simulink subsystem "PowerGain"  (R2023a)
settings: Solver=VariableStepAuto  StartTime=0.0  StopTime=10.0  RelTol=1e-3
model mask{Ku=7.27}
  mask prompts: Ku "Коэффициент усиления"
settings Model: Creator=desire  LastModifiedBy=User

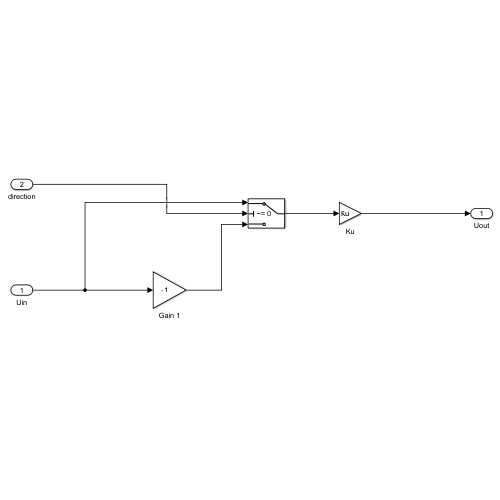
[thumbnail: Simulink's stored preview of the top-level diagram]
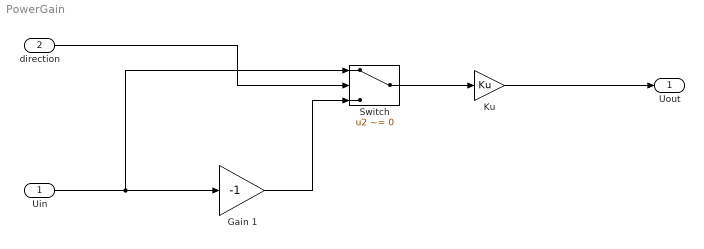
== system PowerGain ==
  Uin : Inport  OutMin=[0]  OutMax=[3.3]
  direction : Inport  Port=2
  Gain 1 : Gain  Gain=-1
  Ku : Gain  Gain=Ku
  Switch : Switch  Criteria=u2 ~= 0  SaturateOnIntegerOverflow=off  InputSameDT=off
  Uout : Outport  OutMin=[0]  OutMax=[24]
  wires:
  Uin/1 -> Switch/1, Gain 1/1
  Gain 1/1 -> Switch/3
  direction/1 -> Switch/2
  Ku/1 -> Uout/1
  Switch/1 -> Ku/1
